simulink library "walk_Gait"  (R2024a)
settings: Solver=VariableStepAuto  StartTime=0.0  StopTime=10.0  RelTol=1e-3
libraries: Plane_Movement_walk_forward x4, delay_and_stop_when_change x3
settings Model: Creator=renre  LastModifiedBy=leona

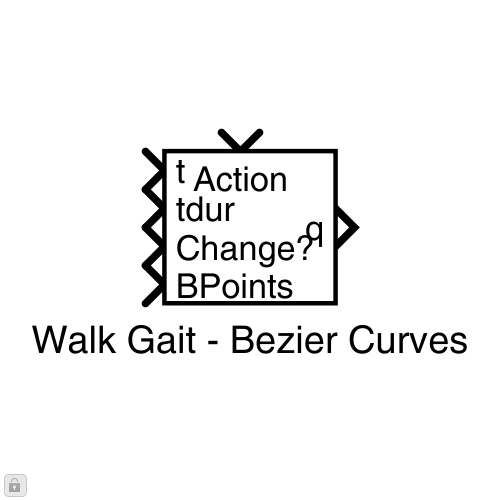
[thumbnail: Simulink's stored preview of the top-level diagram]
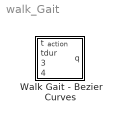
== system walk_Gait ==
  Walk Gait - Bezier Curves : Subsystem

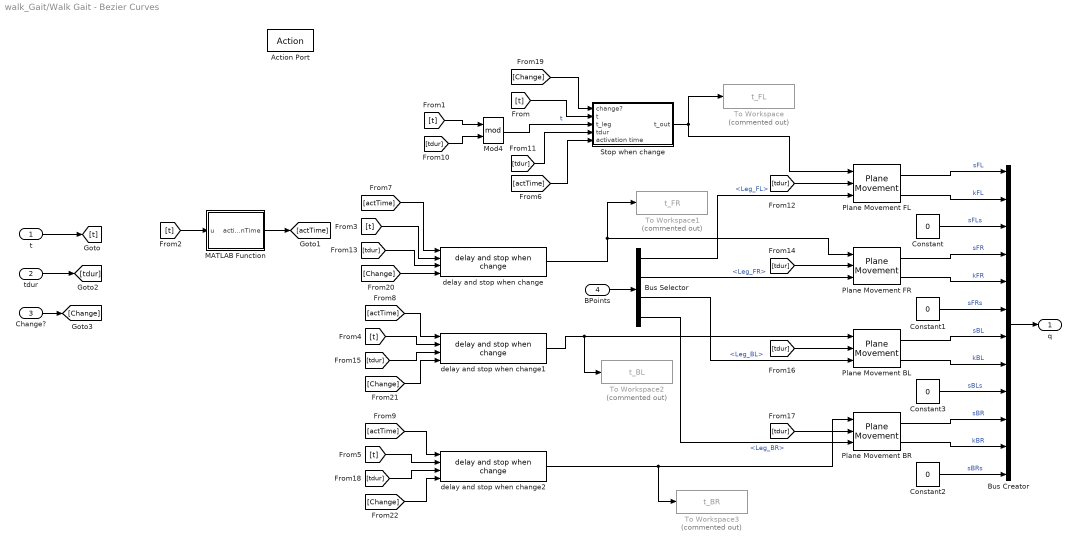
== system walk_Gait/Walk Gait - Bezier Curves ==
  t : Inport
  tdur : Inport  Port=2
  Change? : Inport  Port=3
  BPoints : Inport  Port=4
  Action Port : ActionPort  InitializeStates=reset
  Bus Creator : BusCreator  Inputs=12
  Bus Selector : BusSelector  OutputSignals=Leg_FL,Leg_FR,Leg_BL,Leg_BR
  Constant{,1..3} (4 alike) : Constant  Value=0
  MATLAB Function : MATLAB Function  TreatAsAtomicUnit=on
  Mod4 : Math  Operator=mod
  Plane Movement BL : Plane_Movement_walk_forward/Plane Movement  SystemSampleTime=-1  VariantActivationTime=update diagram  AllowFlexibleInterface=on  Latency=0  AutoFrameSizeCalculation=off
  Plane Movement BR : Plane_Movement_walk_forward/Plane Movement  SystemSampleTime=-1  VariantActivationTime=update diagram  AllowFlexibleInterface=on  Latency=0  AutoFrameSizeCalculation=off
  Plane Movement FL : Plane_Movement_walk_forward/Plane Movement  SystemSampleTime=-1  VariantActivationTime=update diagram  AllowFlexibleInterface=on  Latency=0  AutoFrameSizeCalculation=off
  Plane Movement FR : Plane_Movement_walk_forward/Plane Movement  SystemSampleTime=-1  VariantActivationTime=update diagram  AllowFlexibleInterface=on  Latency=0  AutoFrameSizeCalculation=off
  Stop when change : Subsystem
  To Workspace : ToWorkspace  Commented=on  VariableName=t_FL  SaveFormat=Structure With Time  SampleTime=-1
  To Workspace1 : ToWorkspace  Commented=on  VariableName=t_FR  SaveFormat=Structure  SampleTime=-1
  To Workspace2 : ToWorkspace  Commented=on  VariableName=t_BL  SaveFormat=Structure  SampleTime=-1
  To Workspace3 : ToWorkspace  Commented=on  VariableName=t_BR  SaveFormat=Structure  SampleTime=-1
  delay and stop when change : delay_and_stop_when_change/delay and stop when change  delay=0.5
  delay and stop when change1 : delay_and_stop_when_change/delay and stop when change  delay=0.75
  delay and stop when change2 : delay_and_stop_when_change/delay and stop when change  delay=0.25
  q : Outport
  wires:
  BPoints/1 -> Bus Selector/1
  delay and stop when change1/1 -> To Workspace2/1, Plane Movement BL/1
  delay and stop when change2/1 -> To Workspace3/1, Plane Movement BR/1
  Stop when change/1(t_out) -> Plane Movement FL/1, To Workspace/1
  Change?/1 -> [Change]
  delay and stop when change/1 -> To Workspace1/1, Plane Movement FR/1
  MATLAB Function/1(activationTime) -> [actTime]
  Bus Creator/1 -> q/1
  Plane Movement FL/1 -> Bus Creator/1  "sFL"
  Plane Movement FR/1 -> Bus Creator/4  "sFR"
  Plane Movement FL/2 -> Bus Creator/2  "kFL"
  Plane Movement FR/2 -> Bus Creator/5  "kFR"
  Plane Movement BL/2 -> Bus Creator/8  "kBL"
  Plane Movement BL/1 -> Bus Creator/7  "sBL"
  Plane Movement BR/2 -> Bus Creator/11  "kBR"
  Plane Movement BR/1 -> Bus Creator/10  "sBR"
  t/1 -> [t]
  tdur/1 -> [tdur]
  Mod4/1 -> Stop when change/3(t_leg)  "t"
  Constant/1 -> Bus Creator/3  "sFLs"
  Constant1/1 -> Bus Creator/6  "sFRs"
  Constant3/1 -> Bus Creator/9  "sBLs"
  Constant2/1 -> Bus Creator/12  "sBRs"
  Bus Selector/1 -> Plane Movement FL/3  "<Leg_FL>"
  Bus Selector/2 -> Plane Movement FR/3  "<Leg_FR>"
  Bus Selector/3 -> Plane Movement BL/3  "<Leg_BL>"
  Bus Selector/4 -> Plane Movement BR/3  "<Leg_BR>"
  [t] -> Stop when change/2(t)
  [t] -> Mod4/1
  [t] -> MATLAB Function/1(u)
  [t] -> delay and stop when change/2
  [t] -> delay and stop when change1/2
  [t] -> delay and stop when change2/2
  [actTime] -> Stop when change/5(activation time)
  [actTime] -> delay and stop when change/1
  [actTime] -> delay and stop when change1/1
  [actTime] -> delay and stop when change2/1
  [tdur] -> Mod4/2
  [tdur] -> Stop when change/4(tdur)
  [tdur] -> Plane Movement FL/2
  [tdur] -> delay and stop when change/3
  [tdur] -> Plane Movement FR/2
  [tdur] -> delay and stop when change1/3
  [tdur] -> Plane Movement BL/2
  [tdur] -> Plane Movement BR/2
  [tdur] -> delay and stop when change2/3
  [Change] -> Stop when change/1(change?)
  [Change] -> delay and stop when change/4
  [Change] -> delay and stop when change1/4
  [Change] -> delay and stop when change2/4

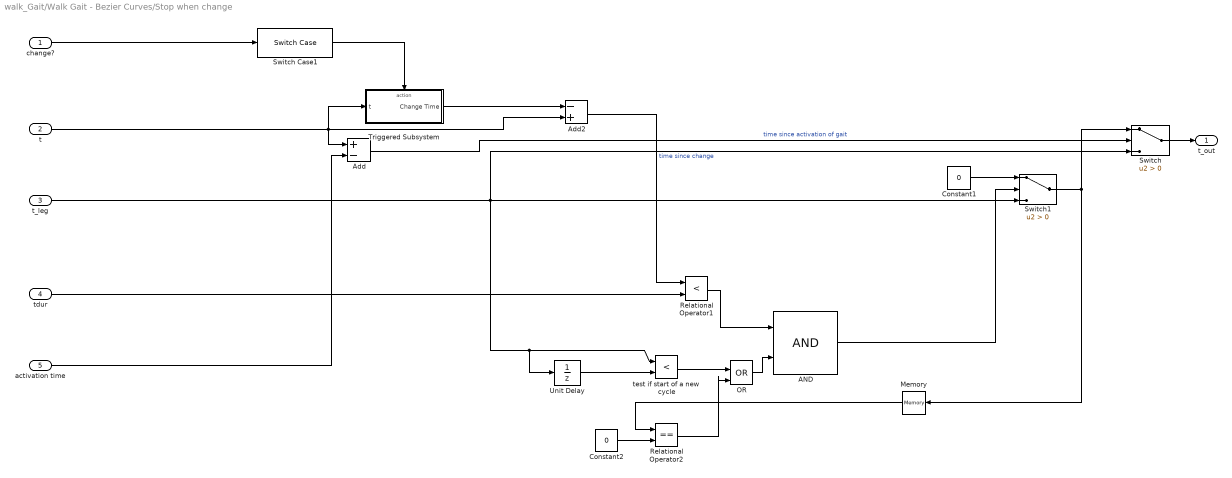
== system walk_Gait/Walk Gait - Bezier Curves/Stop when change ==
  change? : Inport
  t : Inport  Port=2
  t_leg : Inport  Port=3
  tdur : Inport  Port=4
  activation time : Inport  Port=5
  AND : Logic  IconShape=distinctive  AllPortsSameDT=off  OutDataTypeStr=boolean
  Add : Sum  Inputs=+-
  Add2 : Sum  Inputs=-+
  Constant1 : Constant  Value=0
  Constant2 : Constant  Value=0
  Memory : Memory
  OR : Logic  Operator=OR  IconShape=distinctive  AllPortsSameDT=off  OutDataTypeStr=boolean
  Relational Operator1 : RelationalOperator  Operator=<  OutDataTypeStr=boolean  RndMeth=Simplest  InputSameDT=off
  Relational Operator2 : RelationalOperator  Operator===  OutDataTypeStr=boolean  RndMeth=Simplest  InputSameDT=off
  Switch : Switch  Criteria=u2 > Threshold  SaturateOnIntegerOverflow=off  InputSameDT=off
  Switch Case1 : SwitchCase  ShowDefaultCase=off
  Switch1 : Switch  Criteria=u2 > Threshold  SaturateOnIntegerOverflow=off  InputSameDT=off
  Triggered Subsystem : Subsystem  TreatAsAtomicUnit=on
  Unit Delay : UnitDelay  SampleTime=-1  HasFrameUpgradeWarning=on
  test if start of a new cycle : RelationalOperator  Operator=<  OutDataTypeStr=boolean  RndMeth=Simplest  InputSameDT=off
  t_out : Outport
  wires:
  Memory/1 -> Relational Operator2/1
  activation time/1 -> Add/2
  Add/1 -> Switch/2  "time since activation of gait"
  Switch/1 -> t_out/1
  t/1 -> Triggered Subsystem/1(t), Add/1, Add2/2
  Constant1/1 -> Switch1/1
  OR/1 -> AND/2
  Relational Operator2/1 -> OR/2
  tdur/1 -> Relational Operator1/2
  test if start of a new cycle/1 -> OR/1
  Triggered Subsystem/1(Change Time) -> Add2/1
  Constant2/1 -> Relational Operator2/2
  Relational Operator1/1 -> AND/1
  Switch1/1 -> Switch/1, Memory/1
  Unit Delay/1 -> test if start of a new cycle/2
  AND/1 -> Switch1/2
  Switch Case1/1 -> Triggered Subsystem/Action
  change?/1 -> Switch Case1/1
  Add2/1 -> Relational Operator1/1  "time since change"
  t_leg/1 -> test if start of a new cycle/1, Unit Delay/1, Switch1/3, Switch/3

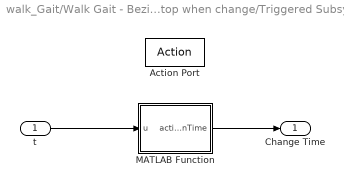
== system walk_Gait/Walk Gait - Bezier Curves/Stop when change/Triggered Subsystem ==
  t : Inport
  Action Port : ActionPort  InitializeStates=reset
  MATLAB Function : MATLAB Function  TreatAsAtomicUnit=on
  Change Time : Outport
  wires:
  t/1 -> MATLAB Function/1(u)
  MATLAB Function/1(activationTime) -> Change Time/1

== matlab function walk_Gait/Walk Gait - Bezier Curves/Stop when change/Triggered Subsystem/MATLAB Function ==
  data: u input; activationTime output
function activationTime = getActivationTime(u)
    persistent t_start
    if isempty(t_start)
        t_start = u;
    end
    activationTime = t_start;
end

== matlab function walk_Gait/Walk Gait - Bezier Curves/MATLAB Function ==
  data: u input; activationTime output
function activationTime = getActivationTime(u)
    persistent t_start
    if isempty(t_start)
        t_start = u;
    end
    activationTime = t_start;
end
